simulink model "Senario_2"  (R2020a)
settings: Solver=VariableStepAuto  StartTime=0.0  StopTime=20.0  RelTol=1e-3
undefined symbols (not defined in the file or in its folder): sigbuilder_block
libraries: fuzblock x2
settings Model: Creator=MANOS  LastModifiedBy=MANOS

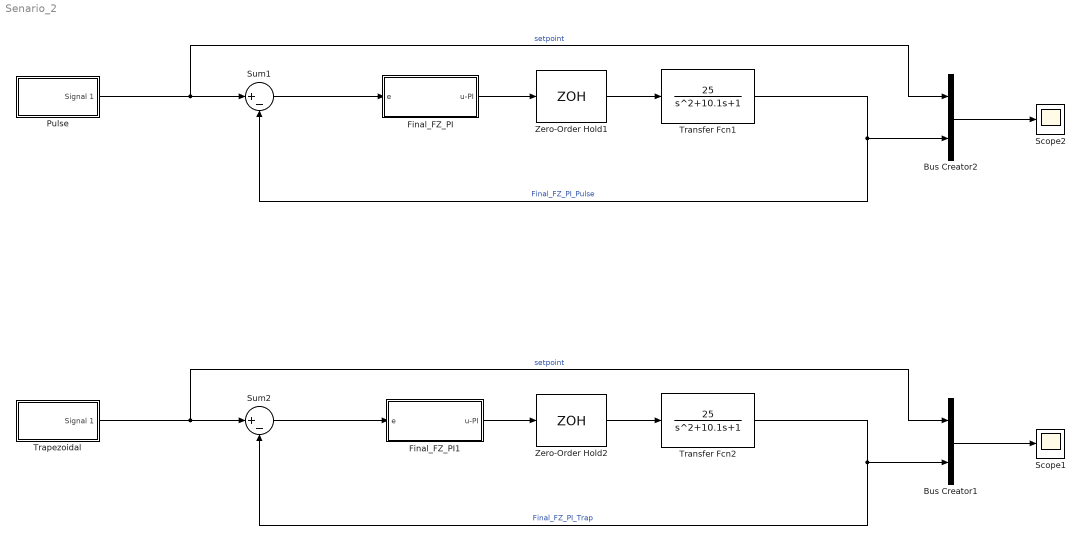
== system Senario_2 ==
  " Pulse" : Subsystem  Tag=STV Subsys  LoadFcn=sigbuilder_block('load');  StartFcn=sigbuilder_block('start');  StopFcn=sigbuilder_block('stop');  ClipboardFcn=sigbuilder_block('clipboard');  mask(Sigbuilder block){tuvar=[0:10]}
      mask help: Simulink:masks:SigbuilderBlock_MD
      mask init:
      | if ~strcmp(get_param(bdroot(gcbh),'SimulationStatus'),'stopped') tuvar = sigbuilder_block('maskInit'); end
      settings: CopyFcn=sigbuilder_block('copy');  DeleteFcn=sigbuilder_block('delete');  ModelCloseFcn=sigbuilder_block('modelClose');  PreSaveFcn=sigbuilder_block('preSave');  PauseFcn=sigbuilder_block('pause');  ContinueFcn=sigbuilder_block('continue');  NameChangeFcn=sigbuilder_block('namechange');  OpenFcn=sigbuilder_block('open',[0.75 5.4 718.5 580.8 ]);  CloseFcn=sigbuilder_block('close');
      mask Display: plot(0, 0, 100, 100,[2, 2, 32, 32, 2], [68, 8, 8, 68, 68],[32, 2], [38, 38], [32, 19, 2],[53, 60, 44], [32, 17, 17, 2],[16, 16, 31, 31]);txt = getActiveGroup(gcbh);text(2, 100, txt,'verticalAlignment', 'top');
  Bus Creator1 : BusCreator  Inputs=2
  Bus Creator2 : BusCreator  Inputs=2
  Final_FZ_PI : Subsystem
  Final_FZ_PI1 : Subsystem
  Scope1 : Scope
  Scope2 : Scope
  Sum1 : Sum  Inputs=|+-
  Sum2 : Sum  Inputs=|+-
  Transfer Fcn1 : TransferFcn  Numerator=[25]  Denominator=[1 10.1 1]
  Transfer Fcn2 : TransferFcn  Numerator=[25]  Denominator=[1 10.1 1]
  Trapezoidal : Subsystem  Tag=STV Subsys  LoadFcn=sigbuilder_block('load');  StartFcn=sigbuilder_block('start');  StopFcn=sigbuilder_block('stop');  ClipboardFcn=sigbuilder_block('clipboard');  mask(Sigbuilder block){tuvar=[0:10]}
      mask help: Simulink:masks:SigbuilderBlock_MD
      mask init:
      | if ~strcmp(get_param(bdroot(gcbh),'SimulationStatus'),'stopped') tuvar = sigbuilder_block('maskInit'); end
      settings: CopyFcn=sigbuilder_block('copy');  DeleteFcn=sigbuilder_block('delete');  ModelCloseFcn=sigbuilder_block('modelClose');  PreSaveFcn=sigbuilder_block('preSave');  PauseFcn=sigbuilder_block('pause');  ContinueFcn=sigbuilder_block('continue');  NameChangeFcn=sigbuilder_block('namechange');  OpenFcn=sigbuilder_block('open',[576.6 36.6 574.8 549.6 ]);  CloseFcn=sigbuilder_block('close');
      mask Display: plot(0, 0, 100, 100,[2, 2, 32, 32, 2], [68, 8, 8, 68, 68],[32, 2], [38, 38], [32, 19, 2],[53, 60, 44], [32, 17, 17, 2],[16, 16, 31, 31]);txt = getActiveGroup(gcbh);text(2, 100, txt,'verticalAlignment', 'top');
  Zero-Order Hold1 : ZeroOrderHold  SampleTime=-1
  Zero-Order Hold2 : ZeroOrderHold  SampleTime=-1
  wires:
  Transfer Fcn1/1 -> Bus Creator2/2, Sum1/2  "Final_FZ_PI_Pulse"
  Sum1/1 -> Final_FZ_PI/1(e)
  " Pulse"/1(Signal 1) -> Bus Creator2/1, Sum1/1  "setpoint"
  Final_FZ_PI/1(u-PI) -> Zero-Order Hold1/1
  Zero-Order Hold1/1 -> Transfer Fcn1/1
  Bus Creator2/1 -> Scope2/1
  Final_FZ_PI1/1(u-PI) -> Zero-Order Hold2/1
  Sum2/1 -> Final_FZ_PI1/1(e)
  Zero-Order Hold2/1 -> Transfer Fcn2/1
  Bus Creator1/1 -> Scope1/1
  Trapezoidal/1(Signal 1) -> Bus Creator1/1, Sum2/1  "setpoint"
  Transfer Fcn2/1 -> Bus Creator1/2, Sum2/2  "Final_FZ_PI_Trap"

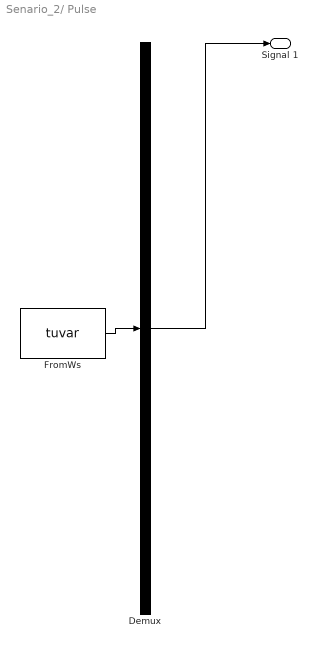
== system Senario_2/ Pulse ==
  Demux : Demux  Tag=STV Demux  Outputs=1
      settings: DisplayOption=none
  FromWs : FromWorkspace  Tag=STV FromWs  VariableName=tuvar
      SigBuilderData=|
      | common.afterFinalStr = 'Extrapolate'
      | common.sampleTime = 0
      | dataSet.timeRange = [0 20]
      | dataSet.name = 'Pulse'
      | sbobj.Groups.Name = 'Pulse'
      | sbobj.Groups.Signals.Name = 'Signal 1'
      | sbobj.Groups.Signals.XData = [0 5 5 10 10 20]
      | sbobj.Groups.Signals.YData = [50 50 20 20 40 40]
      | sbobj.Groups.TimeRange = [0 20]
  Signal 1 : Outport  Tag=STV Outport  VectorParamsAs1DForOutWhenUnconnected=off
  wires:
  Demux/1 -> Signal 1/1
  FromWs/1 -> Demux/1

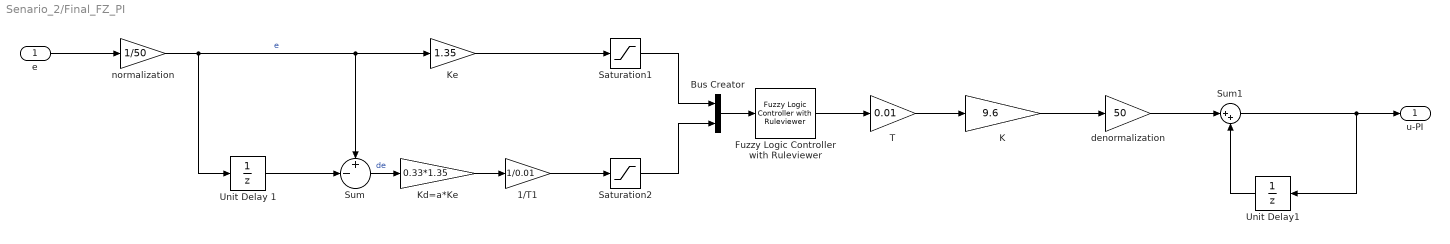
== system Senario_2/Final_FZ_PI ==
  e : Inport
  1/T1 : Gain  Gain=1/0.01
  Bus Creator : BusCreator  Inputs=2
  Fuzzy Logic Controller with Ruleviewer : fuzblock/Fuzzy Logic  Controller  with Ruleviewer  fismatrix=FLC  Ts=2
  K : Gain  Gain=9.6
  Kd=a*Ke : Gain  Gain=0.33*1.35
  Ke : Gain  Gain=1.35
  Saturation1 : Saturate  UpperLimit=1  LowerLimit=-1
  Saturation2 : Saturate  UpperLimit=1  LowerLimit=-1
  Sum : Sum  Inputs=+-|
  Sum1 : Sum  Inputs=|++
  T : Gain  Gain=0.01
  Unit Delay 1 : UnitDelay  SampleTime=-1  HasFrameUpgradeWarning=on
  Unit Delay1 : UnitDelay  SampleTime=-1  HasFrameUpgradeWarning=on
  denormalization : Gain  Gain=50
  normalization : Gain  Gain=1/50
  u-PI : Outport
  wires:
  Unit Delay 1/1 -> Sum/2
  Saturation1/1 -> Bus Creator/1
  Sum/1 -> Kd=a*Ke/1  "de"
  Kd=a*Ke/1 -> 1/T1/1
  denormalization/1 -> Sum1/1
  T/1 -> K/1
  e/1 -> normalization/1
  Ke/1 -> Saturation1/1
  Sum1/1 -> u-PI/1, Unit Delay1/1
  normalization/1 -> Ke/1, Sum/1, Unit Delay 1/1  "e"
  K/1 -> denormalization/1
  1/T1/1 -> Saturation2/1
  Saturation2/1 -> Bus Creator/2
  Bus Creator/1 -> Fuzzy Logic Controller with Ruleviewer/1
  Unit Delay1/1 -> Sum1/2
  Fuzzy Logic Controller with Ruleviewer/1 -> T/1

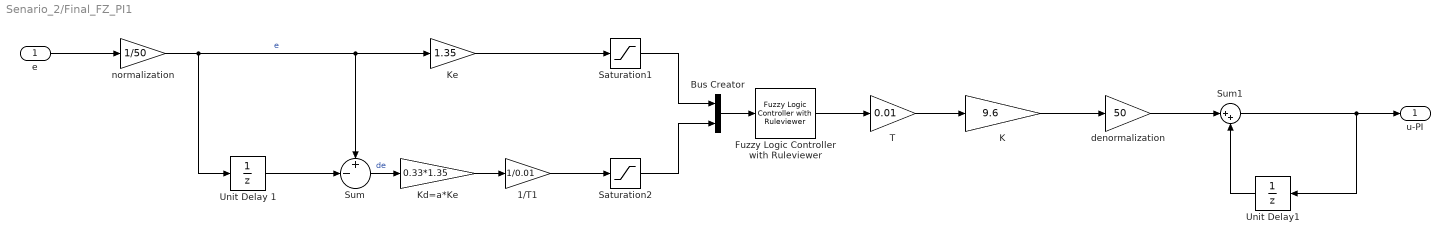
== system Senario_2/Final_FZ_PI1 ==
  e : Inport
  1/T1 : Gain  Gain=1/0.01
  Bus Creator : BusCreator  Inputs=2
  Fuzzy Logic Controller with Ruleviewer : fuzblock/Fuzzy Logic  Controller  with Ruleviewer  fismatrix=FLC  Ts=2
  K : Gain  Gain=9.6
  Kd=a*Ke : Gain  Gain=0.33*1.35
  Ke : Gain  Gain=1.35
  Saturation1 : Saturate  UpperLimit=1  LowerLimit=-1
  Saturation2 : Saturate  UpperLimit=1  LowerLimit=-1
  Sum : Sum  Inputs=+-|
  Sum1 : Sum  Inputs=|++
  T : Gain  Gain=0.01
  Unit Delay 1 : UnitDelay  SampleTime=-1  HasFrameUpgradeWarning=on
  Unit Delay1 : UnitDelay  SampleTime=-1  HasFrameUpgradeWarning=on
  denormalization : Gain  Gain=50
  normalization : Gain  Gain=1/50
  u-PI : Outport
  wires:
  Unit Delay 1/1 -> Sum/2
  Saturation1/1 -> Bus Creator/1
  Sum/1 -> Kd=a*Ke/1  "de"
  Kd=a*Ke/1 -> 1/T1/1
  denormalization/1 -> Sum1/1
  T/1 -> K/1
  e/1 -> normalization/1
  Ke/1 -> Saturation1/1
  Sum1/1 -> u-PI/1, Unit Delay1/1
  normalization/1 -> Ke/1, Sum/1, Unit Delay 1/1  "e"
  K/1 -> denormalization/1
  1/T1/1 -> Saturation2/1
  Saturation2/1 -> Bus Creator/2
  Bus Creator/1 -> Fuzzy Logic Controller with Ruleviewer/1
  Unit Delay1/1 -> Sum1/2
  Fuzzy Logic Controller with Ruleviewer/1 -> T/1

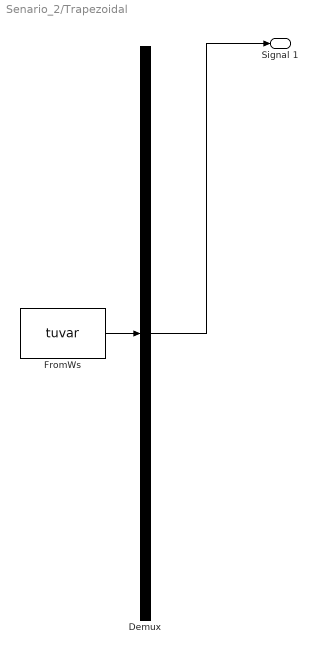
== system Senario_2/Trapezoidal ==
  Demux : Demux  Tag=STV Demux  Outputs=1
      settings: DisplayOption=none
  FromWs : FromWorkspace  Tag=STV FromWs  VariableName=tuvar
      SigBuilderData=|
      | common.afterFinalStr = 'Extrapolate'
      | common.sampleTime = 0
      | dataSet.timeRange = [0 20]
      | dataSet.name = 'Trapezoidal'
      | sbobj.Groups.Name = 'Trapezoidal'
      | sbobj.Groups.Signals.Name = 'Signal 1'
      | sbobj.Groups.Signals.XData = [0 5 10 16 20]
      | sbobj.Groups.Signals.YData = [0 50 49.8 20 0]
      | sbobj.Groups.TimeRange = [0 20]
  Signal 1 : Outport  Tag=STV Outport  VectorParamsAs1DForOutWhenUnconnected=off
  wires:
  Demux/1 -> Signal 1/1
  FromWs/1 -> Demux/1
